simulink model "tanque_area_variavel"  (R2017a)
settings: Solver=ode45  StartTime=0.0  StopTime=40  RelTol=1e-3  EnableMultiTasking=on
InitFcn:
  | clear all
  | clc
  | % Parâmetros do tanque
  | 
  | hM    =  2                       % m
  | B       = 1.5                     % m
  | C       = 4.0                     % m
  | gamma = ((C/2) - (B/2))/hM
  | 
  | rho    = 1000         % kg/m^3
  | g       = 9.8            % m/s^2
  | k       = 0.04
  | 
  | c        = k*sqrt(rho*g)
  | 
  | % Planta
  | 
  | cplanta = 1.1*c
  | 
  | % Condição inicial
  | h0    = 1.5
  | 
  | 
  | %% CONTROLADORES
  | alpha = 1.0 % ponto de linearizacao
  | beta = (pi*gamma^2*(alpha+(B/2)/gamma)^2)
  | 
  | %% SEM AÇÂO INTEGRAL
  | 
  | K_limite_inf = -0.5*c/sqrt(1)
  | % critério tau = 20s
  | K1p = (5/10-1/2*c/(sqrt(alpha)*beta))*beta
  | u_ss = c*sqrt(alpha)
  | 
  | %% COM AÇÃO INTEGRAL
  | %ep = 10
  | %wn  = 6
  | ep  = 5
  | wn  = 6
  | K1pi  =2*ep*wn/beta
  | K2pi = wn^2/beta
  | 
  | ep_desejado = ep
  | ep_real         = (2*ep*wn+c/(sqrt(alpha)*beta))/(2*wn) %devido a influencia do termo desprezado
settings Model: Creator=daniel  LastModifiedBy=daniel
settings DataIOCC: LimitDataPoints=on  SaveFormat=Array
settings OptimizationCC: LifeSpan=inf
settings DebuggingCC: SFUnexpectedBacktrackingDiag=warning  SFNoUnconditionalDefaultTransitionDiag=warning  SFExecutionAtInitializationDiag=none
settings HardwareCC: ProdBitPerPointer=32  ProdBitPerSizeT=32  ProdBitPerPtrDiffT=32  ProdLargestAtomicFloat=None  ProdIntDivRoundTo=Undefined  ProdEndianess=Unspecified  ProdWordSize=32  ProdHWDeviceType=32-bit Generic
settings ModelReferenceCC: PropagateSignalLabelsOutOfModel=off
settings GRTTargetCC: TargetLangStandard=C89/C90 (ANSI)  GeneratePreprocessorConditionals=Disable all
settings ConfigComp: CovMetricSettings=dw  CovHtmlReporting=on  CovSaveCumulativeToWorkspaceVar=on  CovSaveSingleToWorkspaceVar=on  CovExternalEMLEnable=off

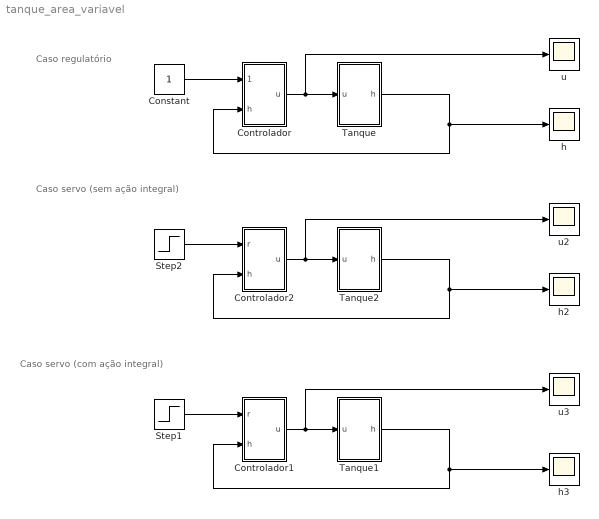
== system tanque_area_variavel ==
  note: Caso regulatório
  note: Caso servo (com ação integral)
  note: Caso servo (sem ação integral)
  Constant : Constant
  Controlador : Subsystem
  Controlador1 : Subsystem
  Controlador2 : Subsystem
  Step1 : Step  Time=25  Before=1  After=1.5  SampleTime=0
  Step2 : Step  Time=25  Before=1  After=1.5  SampleTime=0
  Tanque : Subsystem
  Tanque1 : Subsystem
  Tanque2 : Subsystem
  h : Scope
  h2 : Scope
  h3 : Scope
  u : Scope
  u2 : Scope
  u3 : Scope
  wires:
  Tanque/1(h) -> Controlador/2(h), h/1
  Controlador/1(u) -> u/1, Tanque/1(u)
  Constant/1 -> Controlador/1(alpha)
  Tanque1/1(h) -> Controlador1/2(h), h3/1
  Controlador1/1(u) -> u3/1, Tanque1/1(u)
  Step1/1 -> Controlador1/1(r)
  Tanque2/1(h) -> Controlador2/2(h), h2/1
  Controlador2/1(u) -> u2/1, Tanque2/1(u)
  Step2/1 -> Controlador2/1(r)

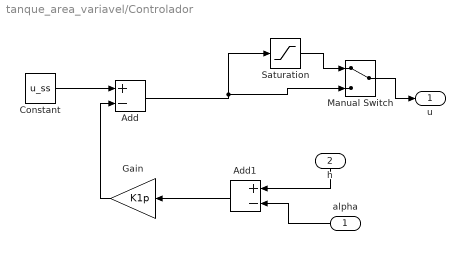
== system tanque_area_variavel/Controlador ==
  alpha : Inport
  h : Inport  Port=2
  Add : Sum  Inputs=+-
  Add1 : Sum  Inputs=+-
  Constant : Constant  Value=u_ss
  Gain : Gain  Gain=K1p
  Manual Switch : ManualSwitch
  Saturation : Saturate  UpperLimit=10  LowerLimit=0
  u : Outport
  wires:
  Gain/1 -> Add/2
  h/1 -> Add1/1
  Add1/1 -> Gain/1
  Saturation/1 -> Manual Switch/1
  Add/1 -> Manual Switch/2, Saturation/1
  Manual Switch/1 -> u/1
  alpha/1 -> Add1/2
  Constant/1 -> Add/1

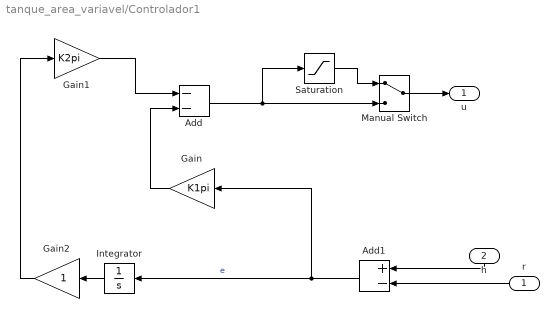
== system tanque_area_variavel/Controlador1 ==
  r : Inport
  h : Inport  Port=2
  Add : Sum  Inputs=--
  Add1 : Sum  Inputs=+-
  Gain : Gain  Gain=K1pi
  Gain1 : Gain  Gain=K2pi
  Gain2 : Gain
  Integrator : Integrator  InitialCondition=h0-1
  Manual Switch : ManualSwitch
  Saturation : Saturate  UpperLimit=10  LowerLimit=0
  u : Outport
  wires:
  Gain1/1 -> Add/1
  Gain/1 -> Add/2
  h/1 -> Add1/1
  r/1 -> Add1/2
  Saturation/1 -> Manual Switch/1
  Add1/1 -> Gain/1, Integrator/1  "e"
  Gain2/1 -> Gain1/1
  Integrator/1 -> Gain2/1
  Add/1 -> Manual Switch/2, Saturation/1
  Manual Switch/1 -> u/1

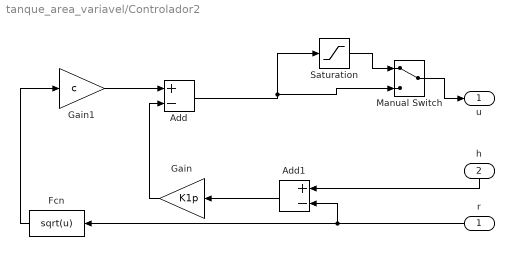
== system tanque_area_variavel/Controlador2 ==
  r : Inport
  h : Inport  Port=2
  Add : Sum  Inputs=+-
  Add1 : Sum  Inputs=+-
  Fcn : Fcn  Expr=sqrt(u)
  Gain : Gain  Gain=K1p
  Gain1 : Gain  Gain=c
  Manual Switch : ManualSwitch
  Saturation : Saturate  UpperLimit=10  LowerLimit=0
  u : Outport
  wires:
  Gain/1 -> Add/2
  h/1 -> Add1/1
  Add1/1 -> Gain/1
  Saturation/1 -> Manual Switch/1
  Add/1 -> Manual Switch/2, Saturation/1
  Manual Switch/1 -> u/1
  r/1 -> Fcn/1, Add1/2
  Gain1/1 -> Add/1
  Fcn/1 -> Gain1/1

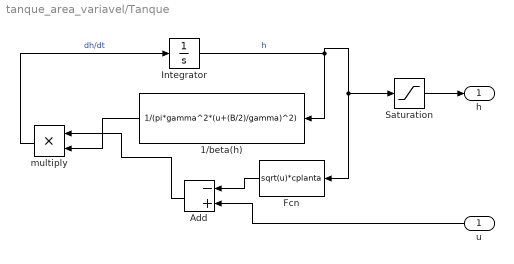
== system tanque_area_variavel/Tanque ==
  u : Inport
  1/beta(h) : Fcn  Expr=1/(pi*gamma^2*(u+(B/2)/gamma)^2)
  Add : Sum  Inputs=-+
  Fcn : Fcn  Expr=sqrt(u)*cplanta
  Integrator : Integrator  InitialCondition=h0
  Saturation : Saturate  UpperLimit=hM  LowerLimit=0
  multiply : Product  Inputs=**
  h : Outport
  wires:
  Integrator/1 -> Saturation/1, Fcn/1, 1/beta(h)/1  "h"
  Saturation/1 -> h/1
  Fcn/1 -> Add/1
  1/beta(h)/1 -> multiply/2
  Add/1 -> multiply/1
  u/1 -> Add/2
  multiply/1 -> Integrator/1  "dh/dt"

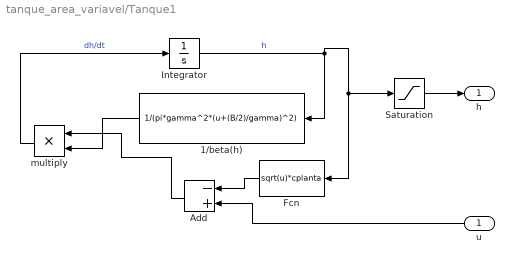
== system tanque_area_variavel/Tanque1 ==
  u : Inport
  1/beta(h) : Fcn  Expr=1/(pi*gamma^2*(u+(B/2)/gamma)^2)
  Add : Sum  Inputs=-+
  Fcn : Fcn  Expr=sqrt(u)*cplanta
  Integrator : Integrator  InitialCondition=h0
  Saturation : Saturate  UpperLimit=hM  LowerLimit=0
  multiply : Product  Inputs=**
  h : Outport
  wires:
  Integrator/1 -> Saturation/1, Fcn/1, 1/beta(h)/1  "h"
  Saturation/1 -> h/1
  Fcn/1 -> Add/1
  1/beta(h)/1 -> multiply/2
  Add/1 -> multiply/1
  u/1 -> Add/2
  multiply/1 -> Integrator/1  "dh/dt"

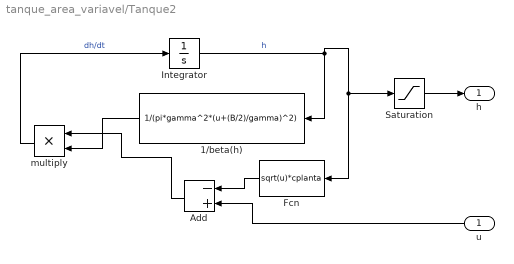
== system tanque_area_variavel/Tanque2 ==
  u : Inport
  1/beta(h) : Fcn  Expr=1/(pi*gamma^2*(u+(B/2)/gamma)^2)
  Add : Sum  Inputs=-+
  Fcn : Fcn  Expr=sqrt(u)*cplanta
  Integrator : Integrator  InitialCondition=h0
  Saturation : Saturate  UpperLimit=hM  LowerLimit=0
  multiply : Product  Inputs=**
  h : Outport
  wires:
  Integrator/1 -> Saturation/1, Fcn/1, 1/beta(h)/1  "h"
  Saturation/1 -> h/1
  Fcn/1 -> Add/1
  1/beta(h)/1 -> multiply/2
  Add/1 -> multiply/1
  u/1 -> Add/2
  multiply/1 -> Integrator/1  "dh/dt"
